simulink model "Copter"  (R2025a)
settings: Solver=ode1  StartTime=0.0  StopTime=inf  FixedStep=0.00125  RelTol=1e-3
libraries: aerolib6dof2 x4, AP_Conector_new x4
settings Model: PauseTimes=0:1  Creator=Peter  LastModifiedBy=danie
settings SolverCC: NumberNewtonIterations=2.0  AlgebraicLoopSolver=TrustRegion
settings DebuggingCC: UnconnectedInputMsg=warning  UnconnectedOutputMsg=warning  UnconnectedLineMsg=warning
settings ModelReferenceCC: EnableRefExpFcnMdlSchedulingChecks=on
settings RTWCC: GPUComputeCapability=3.5

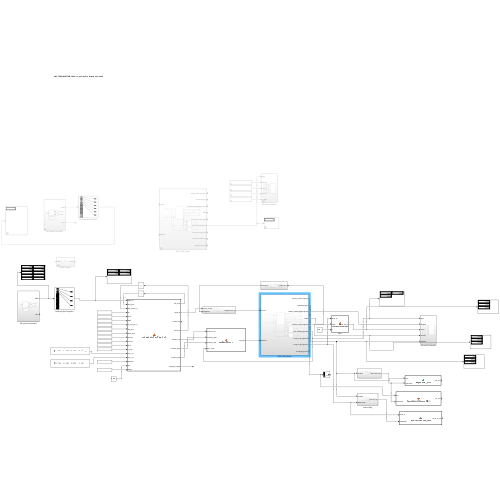
[thumbnail: Simulink's stored preview of the top-level diagram]
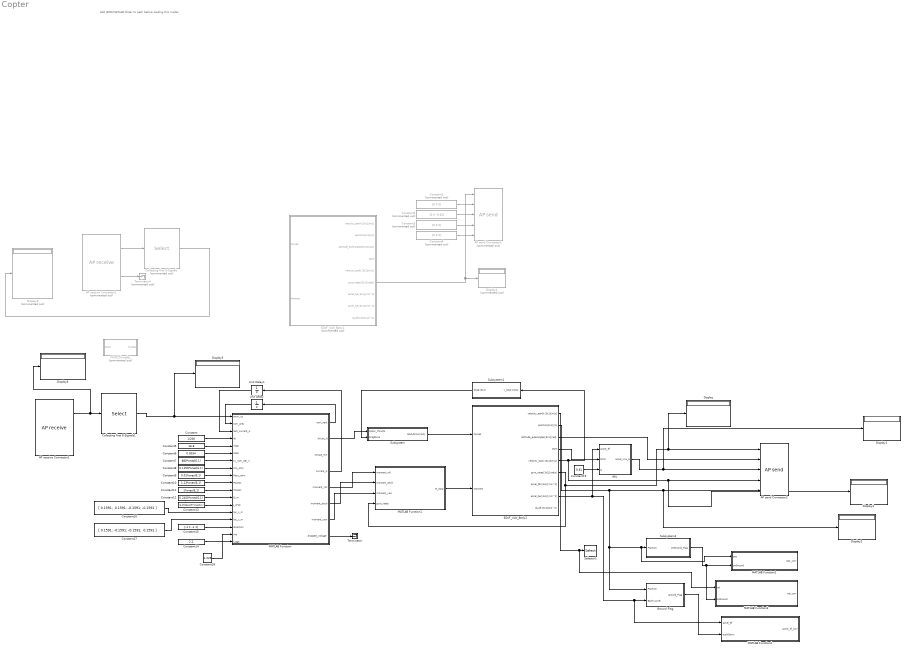
== system Copter ==
  note: Add JSON/MATLAB folder to path before loading this model
  6DoF_UAV_Body1 : Subsystem  Commented=on
  6DoF_UAV_Body2 : Subsystem
  AP receive Connector1 : AP_Conector_new/AP receive  Commented=on  SystemSampleTime=-1  VariantActivationTime=update diagram  EmptyChoice=off  PassThrough=off  PassThroughVariantControl=(default)  EmptyChoiceVariantControl=(default)  AllowFlexibleInterface=on  Latency=0  AutoFrameSizeCalculation=off
  AP receive Connector2 : AP_Conector_new/AP receive  SystemSampleTime=-1  VariantActivationTime=update diagram  EmptyChoice=off  PassThrough=off  PassThroughVariantControl=(default)  EmptyChoiceVariantControl=(default)  AllowFlexibleInterface=on  Latency=0  AutoFrameSizeCalculation=off
  AP send Connector1 : AP_Conector_new/AP send  Commented=on  SystemSampleTime=-1  VariantActivationTime=update diagram  EmptyChoice=off  PassThrough=off  PassThroughVariantControl=(default)  EmptyChoiceVariantControl=(default)  AllowFlexibleInterface=on  Latency=0  AutoFrameSizeCalculation=off
  AP send Connector2 : AP_Conector_new/AP send  SystemSampleTime=-1  VariantActivationTime=update diagram  EmptyChoice=off  PassThrough=off  PassThroughVariantControl=(default)  EmptyChoiceVariantControl=(default)  AllowFlexibleInterface=on  Latency=0  AutoFrameSizeCalculation=off
  Collecting first 6-Signals : Selector  Commented=on  InputPortWidth=16  IndexOptions=Index vector (dialog)  Indices=[1 2 3 4 5 6]  OutputSizes=1
  Collecting first 6-Signals1 : Selector  InputPortWidth=16  IndexOptions=Index vector (dialog)  Indices=[1 2 3 4]  OutputSizes=1
  Constant : Constant  Value=1/200
  Constant1 : Constant  Commented=on  Value=[0 0 0]
  Constant10 : Constant  Value=1.13*ones(6,1)
  Constant11 : Constant  Value=1*ones(6,1)
  Constant12 : Constant  Value=0.2450*ones(6,1)
  Constant13 : Constant  Value=(6.2526e-05)*ones(6,1)
  Constant14 : Constant  Value=2.2
  Constant15 : Constant  Value=[-1 1 -1 1]
  Constant16 : Constant  Value="[ 0.1591;  0.1591; -0.1591; -0.1591 ]"
  Constant17 : Constant  Value="[ 0.1591; -0.1591; -0.1591;  0.1591 ]"
  Constant18 : Constant  Value=1.225
  Constant19 : Constant  Value=9.81
  Constant2 : Constant  Commented=on  Value=[0 0 -9.81]
  Constant3 : Constant  Commented=on  Value=[0 0 0]
  Constant4 : Constant  Commented=on  Value=[0 0 0]
  Constant5 : Constant  Value=16.8
  Constant6 : Constant  Value=0.0034
  Constant7 : Constant  Value=880*ones(6,1)
  Constant8 : Constant  Value=0.1150*ones(6,1)
  Constant9 : Constant  Value=0.01*ones(6,1)
  Display{,1..3,5..6} (6 alike) : Display
  Display4 : Display  Commented=on
  Display9 : Display  Commented=on
  Ground Flag : Subsystem
  IMU : MATLAB Function  TreatAsAtomicUnit=on
  MATLAB Function : MATLAB Function  TreatAsAtomicUnit=on
  MATLAB Function1 : MATLAB Function  TreatAsAtomicUnit=on
  MATLAB Function2 : MATLAB Function  TreatAsAtomicUnit=on
  MATLAB Function3 : MATLAB Function  TreatAsAtomicUnit=on
  MATLAB Function4 : MATLAB Function  TreatAsAtomicUnit=on
  PWM2Throttle1 : Subsystem  Commented=on
  Selector1 : Selector  InputPortWidth=3  IndexOptions=Index vector (dialog)  Indices=[3]  OutputSizes=1
  Subsystem : Subsystem
  Subsystem1 : Subsystem
  Subsystem2 : Subsystem
  Terminator : Terminator
  Terminator4 : Terminator  Commented=on
  Unit Delay : UnitDelay  SampleTime=-1  HasFrameUpgradeWarning=on
  Unit Delay1 : UnitDelay  SampleTime=-1  HasFrameUpgradeWarning=on
  wires:
  Constant1/1 -> AP send Connector1/2
  Constant4/1 -> AP send Connector1/5
  Constant3/1 -> AP send Connector1/4
  Constant2/1 -> AP send Connector1/3
  AP receive Connector1/1 -> Collecting first 6-Signals/1
  AP receive Connector1/2 -> Terminator4/1
  Collecting first 6-Signals/1 -> Display9/1
  6DoF_UAV_Body1/6(gyro_rates[3x1][rad/s]) -> Display4/1, AP send Connector1/1
  MATLAB Function/1(rpm_next) -> Unit Delay/1
  Unit Delay/1 -> MATLAB Function/2(rpm_prev)
  AP receive Connector2/1 -> Display6/1, Collecting first 6-Signals1/1
  Constant/1 -> MATLAB Function/4(dt)
  Constant5/1 -> MATLAB Function/5(Vbat)
  Constant6/1 -> MATLAB Function/6(Rbat)
  Constant7/1 -> MATLAB Function/7(kv_rpm_per_V)
  Constant8/1 -> MATLAB Function/8(Rm_ohm)
  Constant9/1 -> MATLAB Function/9(Resc_ohm)
  Constant11/1 -> MATLAB Function/11(TConst)
  Constant10/1 -> MATLAB Function/10(PConst)
  Constant12/1 -> MATLAB Function/12(D_m)
  Constant13/1 -> MATLAB Function/13(J_prop)
  Constant14/1 -> MATLAB Function/18(fudge)
  MATLAB Function/4(current_A) -> Unit Delay1/1
  Unit Delay1/1 -> MATLAB Function/3(last_current_A)
  Constant15/1 -> MATLAB Function/16(direction)
  Constant16/1 -> MATLAB Function/14(loc_x_m)
  Constant17/1 -> MATLAB Function/15(loc_y_m)
  MATLAB Function/8(dropped_voltage) -> Terminator/1
  MATLAB Function/2(thrust_N) -> Subsystem/1(Motor_thrusts)
  Subsystem/1(Bodyforce [3x1]) -> 6DoF_UAV_Body2/1(Forces)
  6DoF_UAV_Body2/5(velocity_body [3x1][m/s]) -> Display3/1, AP send Connector2/4, Subsystem1/1(v_body [3x1])
  Subsystem1/1(Drag [3x1]) -> Subsystem/2(Dragforce)
  Constant18/1 -> MATLAB Function/17(rho)
  MATLAB Function1/1(M_body) -> 6DoF_UAV_Body2/2(Moment)
  MATLAB Function/5(moment_roll) -> MATLAB Function1/1(moment_roll)
  MATLAB Function/6(moment_pitch) -> MATLAB Function1/2(moment_pitch)
  MATLAB Function/7(moment_yaw) -> MATLAB Function1/3(moment_yaw)
  6DoF_UAV_Body2/6(gyro_rates[3x1][rad/s]) -> Display/1, AP send Connector2/1, MATLAB Function1/4(gyro_rates)
  6DoF_UAV_Body2/4(DCM) -> IMU/2(DCM)
  Constant19/1 -> IMU/3(g)
  6DoF_UAV_Body2/8(accel_be [3x1][m/s^2]) -> MATLAB Function4/1(accel_ef), Ground Flag/2(Earth Accel), IMU/1(accel_ef)
  IMU/1(accel_imu_b) -> Display1/1, AP send Connector2/3
  6DoF_UAV_Body2/3(attitude_eulerangles[3x1][rad]) -> AP send Connector2/2
  Collecting first 6-Signals1/1 -> Display5/1, MATLAB Function/1(pwm_us)
  6DoF_UAV_Body2/1(velocity_earth [3x1][m/s]) -> MATLAB Function3/1(vel), Selector1/1
  Ground Flag/1(ground_Flag) -> MATLAB Function4/2(pushDown)
  6DoF_UAV_Body2/2(position[3x1][m]) -> Ground Flag/1(Position), MATLAB Function2/1(pos), Subsystem2/1(Position), Display2/1, AP send Connector2/5
  Subsystem2/1(onGround_Flag) -> MATLAB Function3/2(onGround), MATLAB Function2/2(onGround)

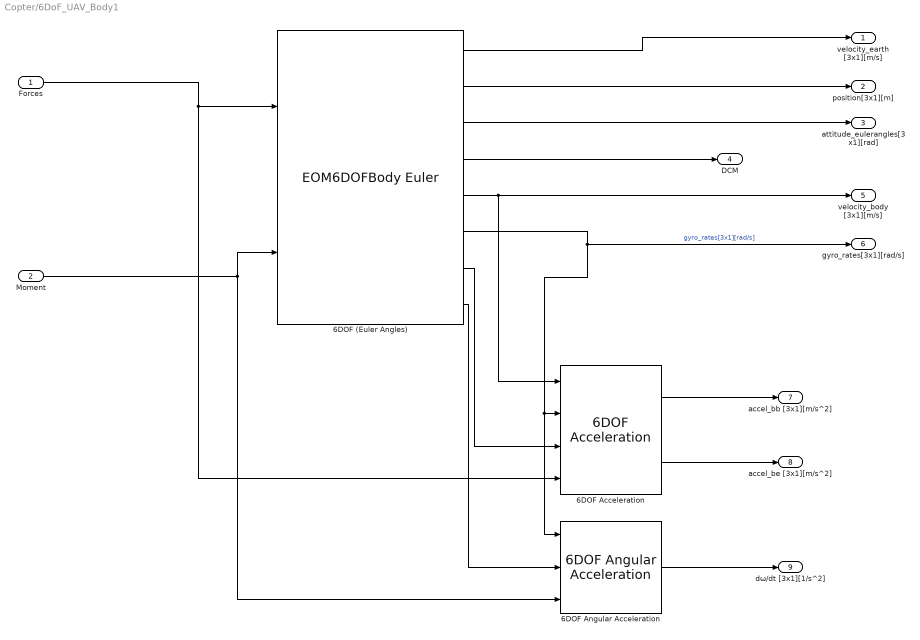
== system Copter/6DoF_UAV_Body1 ==
  Forces : Inport
  Moment : Inport  Port=2
  6DOF (Euler Angles) : EOM6DOFBodyEuler  mass_0=parameters.m  inertia=parameters.I  mass_flag=on
  6DOF Acceleration : aerolib6dof2/6DOF Acceleration  units=Metric (MKS)  mtype=Fixed  vre_flag=off
  6DOF Angular Acceleration : aerolib6dof2/6DOF Angular Acceleration  units=Metric (MKS)  mtype=Fixed
  velocity_earth [3x1][m/s] : Outport
  position[3x1][m] : Outport  Port=2
  attitude_eulerangles[3x1][rad] : Outport  Port=3
  DCM : Outport  Port=4
  velocity_body [3x1][m/s] : Outport  Port=5
  gyro_rates[3x1][rad/s] : Outport  Port=6
  accel_bb [3x1][m/s^2] : Outport  Port=7
  accel_be [3x1][m/s^2] : Outport  Port=8
  dω/dt [3x1][1/s^2] : Outport  Port=9
  wires:
  6DOF (Euler Angles)/3 -> attitude_eulerangles[3x1][rad]/1
  Moment/1 -> 6DOF (Euler Angles)/2, 6DOF Angular Acceleration/3
  6DOF Angular Acceleration/1 -> dω/dt [3x1][1/s^2]/1
  6DOF (Euler Angles)/6 -> gyro_rates[3x1][rad/s]/1, 6DOF Angular Acceleration/1, 6DOF Acceleration/2  "gyro_rates[3x1][rad/s]"
  6DOF Acceleration/2 -> accel_be [3x1][m/s^2]/1
  6DOF (Euler Angles)/5 -> velocity_body [3x1][m/s]/1, 6DOF Acceleration/1
  6DOF Acceleration/1 -> accel_bb [3x1][m/s^2]/1
  6DOF (Euler Angles)/8 -> 6DOF Angular Acceleration/2
  6DOF (Euler Angles)/7 -> 6DOF Acceleration/3
  6DOF (Euler Angles)/2 -> position[3x1][m]/1
  Forces/1 -> 6DOF Acceleration/4, 6DOF (Euler Angles)/1
  6DOF (Euler Angles)/1 -> velocity_earth [3x1][m/s]/1
  6DOF (Euler Angles)/4 -> DCM/1

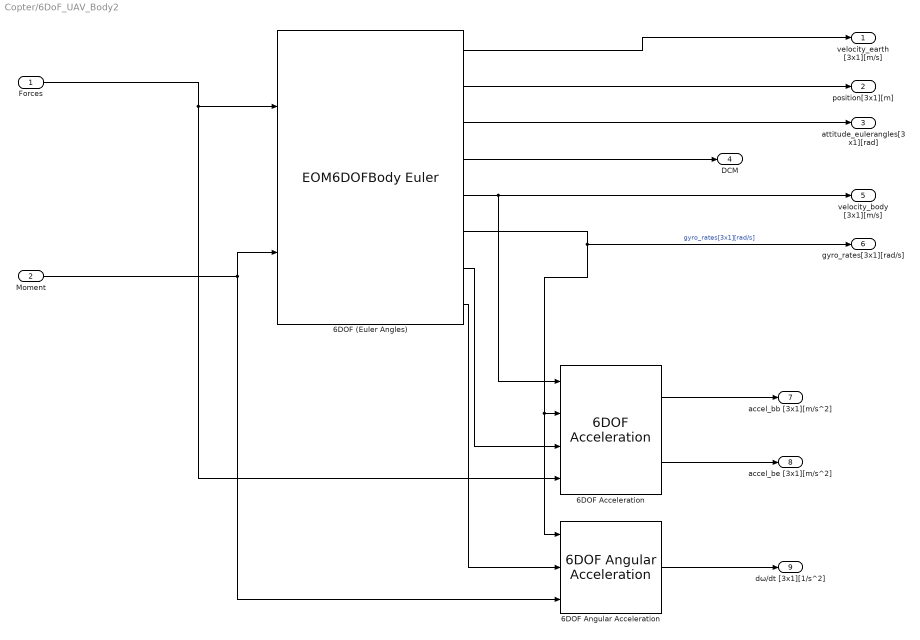
== system Copter/6DoF_UAV_Body2 ==
  Forces : Inport
  Moment : Inport  Port=2
  6DOF (Euler Angles) : EOM6DOFBodyEuler  mass_0=2  inertia=diag([0.0065 0.0065 0.0065])  mass_flag=on
  6DOF Acceleration : aerolib6dof2/6DOF Acceleration  units=Metric (MKS)  mtype=Fixed  vre_flag=off
  6DOF Angular Acceleration : aerolib6dof2/6DOF Angular Acceleration  units=Metric (MKS)  mtype=Fixed
  velocity_earth [3x1][m/s] : Outport
  position[3x1][m] : Outport  Port=2
  attitude_eulerangles[3x1][rad] : Outport  Port=3
  DCM : Outport  Port=4
  velocity_body [3x1][m/s] : Outport  Port=5
  gyro_rates[3x1][rad/s] : Outport  Port=6
  accel_bb [3x1][m/s^2] : Outport  Port=7
  accel_be [3x1][m/s^2] : Outport  Port=8
  dω/dt [3x1][1/s^2] : Outport  Port=9
  wires:
  6DOF (Euler Angles)/4 -> DCM/1
  6DOF (Euler Angles)/1 -> velocity_earth [3x1][m/s]/1
  Forces/1 -> 6DOF (Euler Angles)/1, 6DOF Acceleration/4
  6DOF (Euler Angles)/2 -> position[3x1][m]/1
  6DOF (Euler Angles)/7 -> 6DOF Acceleration/3
  6DOF (Euler Angles)/8 -> 6DOF Angular Acceleration/2
  6DOF Acceleration/1 -> accel_bb [3x1][m/s^2]/1
  6DOF (Euler Angles)/5 -> 6DOF Acceleration/1, velocity_body [3x1][m/s]/1
  6DOF Acceleration/2 -> accel_be [3x1][m/s^2]/1
  6DOF (Euler Angles)/6 -> 6DOF Acceleration/2, 6DOF Angular Acceleration/1, gyro_rates[3x1][rad/s]/1  "gyro_rates[3x1][rad/s]"
  6DOF Angular Acceleration/1 -> dω/dt [3x1][1/s^2]/1
  Moment/1 -> 6DOF Angular Acceleration/3, 6DOF (Euler Angles)/2
  6DOF (Euler Angles)/3 -> attitude_eulerangles[3x1][rad]/1

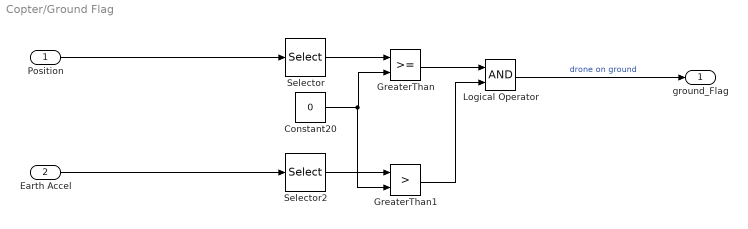
== system Copter/Ground Flag ==
  Position : Inport
  Earth Accel : Inport  Port=2
  Constant20 : Constant  Value=0
  GreaterThan : RelationalOperator  OutDataTypeStr=boolean  RndMeth=Simplest  InputSameDT=off
  GreaterThan1 : RelationalOperator  Operator=>  OutDataTypeStr=boolean  RndMeth=Simplest  InputSameDT=off
  Logical Operator : Logic  AllPortsSameDT=off  OutDataTypeStr=boolean
  Selector : Selector  InputPortWidth=3  IndexOptions=Index vector (dialog)  Indices=[3]  OutputSizes=1
  Selector2 : Selector  InputPortWidth=3  IndexOptions=Index vector (dialog)  Indices=[3]  OutputSizes=1
  ground_Flag : Outport
  wires:
  Selector2/1 -> GreaterThan1/1
  Selector/1 -> GreaterThan/1
  Constant20/1 -> GreaterThan1/2, GreaterThan/2
  Logical Operator/1 -> ground_Flag/1  "drone on ground"
  GreaterThan/1 -> Logical Operator/1
  GreaterThan1/1 -> Logical Operator/2
  Earth Accel/1 -> Selector2/1
  Position/1 -> Selector/1

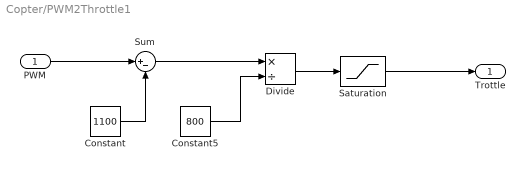
== system Copter/PWM2Throttle1 ==
  PWM : Inport
  Constant : Constant  Value=1100
  Constant5 : Constant  Value=800
  Divide : Product  Inputs=*/
  Saturation : Saturate  UpperLimit=1  LowerLimit=0
  Sum : Sum  Inputs=|+-
  Trottle : Outport
  wires:
  PWM/1 -> Sum/1
  Constant5/1 -> Divide/2
  Sum/1 -> Divide/1
  Divide/1 -> Saturation/1
  Constant/1 -> Sum/2
  Saturation/1 -> Trottle/1

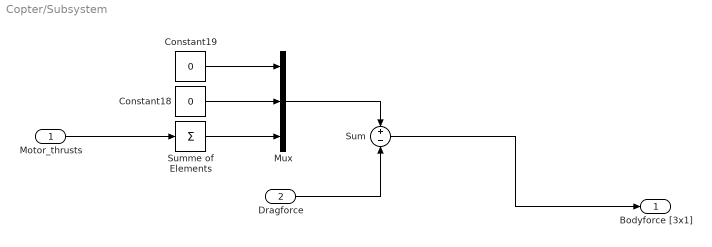
== system Copter/Subsystem ==
  Motor_thrusts : Inport
  Dragforce : Inport  Port=2
  Constant18 : Constant  Value=0
  Constant19 : Constant  Value=0
  Mux : Mux  Inputs=3
  Sum : Sum  Inputs=+-
  Summe of Elements : Sum  Inputs=+
  Bodyforce [3x1] : Outport
  wires:
  Constant19/1 -> Mux/1
  Sum/1 -> Bodyforce [3x1]/1
  Motor_thrusts/1 -> Summe of Elements/1
  Mux/1 -> Sum/1
  Dragforce/1 -> Sum/2
  Constant18/1 -> Mux/2
  Summe of Elements/1 -> Mux/3

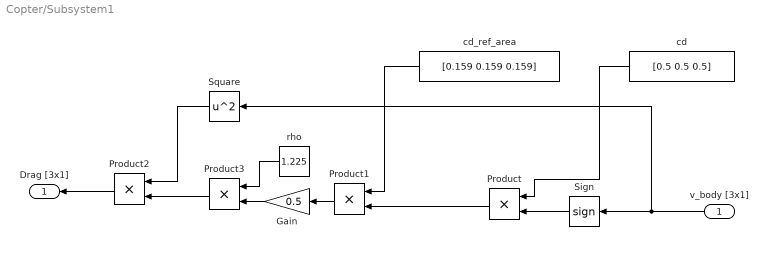
== system Copter/Subsystem1 ==
  v_body [3x1] : Inport
  Gain : Gain  Gain=0.5
  Product{,1..3} (4 alike) : Product
  Sign : Signum
  Square : Math  Operator=square
  cd : Constant  Value=[0.5 0.5 0.5]
  cd_ref_area : Constant  Value=[0.159 0.159 0.159]
  rho : Constant  Value=1.225
  Drag [3x1] : Outport
  wires:
  rho/1 -> Product3/1
  Gain/1 -> Product3/2
  Square/1 -> Product2/1
  cd/1 -> Product/1
  Product3/1 -> Product2/2
  v_body [3x1]/1 -> Square/1, Sign/1
  Sign/1 -> Product/2
  cd_ref_area/1 -> Product1/1
  Product/1 -> Product1/2
  Product1/1 -> Gain/1
  Product2/1 -> Drag [3x1]/1

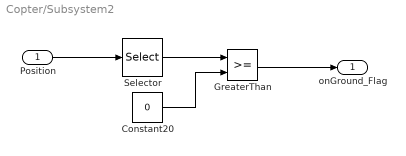
== system Copter/Subsystem2 ==
  Position : Inport
  Constant20 : Constant  Value=0
  GreaterThan : RelationalOperator  OutDataTypeStr=boolean  RndMeth=Simplest  InputSameDT=off
  Selector : Selector  InputPortWidth=3  IndexOptions=Index vector (dialog)  Indices=[3]  OutputSizes=1
  onGround_Flag : Outport
  wires:
  Constant20/1 -> GreaterThan/2
  GreaterThan/1 -> onGround_Flag/1
  Position/1 -> Selector/1
  Selector/1 -> GreaterThan/1

== matlab function Copter/MATLAB Function1 ==
  data: moment_roll input; M_body output; moment_pitch input; moment_yaw input; gyro_rates input
function M_body = buildBodyMoments(moment_roll, moment_pitch, moment_yaw, gyro_rates)
%#codegen
% moment_roll  [Mx1]  = T_i * x_i
% moment_pitch [Mx1]  = T_i * y_i
% moment_yaw   [Mx1]  = -Q_i * dir_i
% gyro_rates   [3x1]  = [p;q;r] rad/s (optional, for rotational drag)

% --- Sum motor contributions (SCRIPT-KONFORM)
Mx = -sum(moment_roll);
My =  sum(moment_pitch);
Mz =  sum(moment_yaw);

M_body = [Mx; My; Mz];

% --- Optional: rotational drag (wie im Script)
% rotational_drag = 0.2 * sign(gyro) .* gyro.^2;
if ~isempty(gyro_rates)
    rot_drag = 0.2 * sign(gyro_rates) .* (gyro_rates.^2);
    M_body = M_body - rot_drag;
end

end

== matlab function Copter/MATLAB Function ==
  data: pwm_us input; rpm_next output; rpm_prev input; last_current_A input; dt input; Vbat input; Rbat input; kv_rpm_per_V input; Rm_ohm input; Resc_ohm input; PConst input; TConst input; D_m input; J_prop input; loc_x_m input; loc_y_m input; direction input; rho input; fudge input; thrust_N output; torque_Nm output; current_A output; moment_roll output; moment_pitch output; moment_yaw output; dropped_voltage output
function [rpm_next, thrust_N, torque_Nm, current_A, ...
          moment_roll, moment_pitch, moment_yaw, dropped_voltage] = ...
    motorActuationFromPWM_1to1(pwm_us, rpm_prev, last_current_A, dt, ...
    Vbat, Rbat, ...
    kv_rpm_per_V, Rm_ohm, Resc_ohm, ...
    PConst, TConst, D_m, J_prop, ...
    loc_x_m, loc_y_m, direction, ...
    rho, fudge)
%#codegen
% 1:1 Logik wie im Jason/Hexsoon physics_step Motor-Loop

M = numel(pwm_us);

% Prealloc
rpm_next     = zeros(size(pwm_us));
thrust_N     = zeros(size(pwm_us));
torque_Nm    = zeros(size(pwm_us));
current_A    = zeros(size(pwm_us));
moment_roll  = zeros(size(pwm_us));
moment_pitch = zeros(size(pwm_us));
moment_yaw   = zeros(size(pwm_us));

% --- Battery sag (current draw from last step)
I_total = 0.0;
for i = 1:M
    I_total = I_total + last_current_A(i);
end
dropped_voltage = Vbat - Rbat * I_total;

% (Script macht keinen clamp; optional nur, wenn nötig)
% if dropped_voltage < 0, dropped_voltage = 0; end

two_pi = 2.0*pi;

for i = 1:M
    % --- throttle (0..1) from PWM
    throttle = (pwm_us(i) - 1100.0) / 800.0;
    if throttle < 0.0
        throttle = 0.0;
    elseif throttle > 1.0
        throttle = 1.0;
    end

    % effective voltage
    voltage = throttle * dropped_voltage;

    % Kt = 1 / (kv * (2*pi/60))
    kv = kv_rpm_per_V(i);
    if kv <= 1e-6
        kv = 1e-6;
    end
    Kt = 1.0 / (kv * (two_pi/60.0));

    % current = ((kv*voltage) - rpm) / ((Rtot)*kv)
    Rtot = Rm_ohm(i) + Resc_ohm(i);
    if Rtot <= 1e-6
        Rtot = 1e-6;
    end
    current = ((kv * voltage) - rpm_prev(i)) / (Rtot * kv);

    % torque = current * Kt
    torque = current * Kt;

    % prop_drag = PConst * rho * (rpm/60)^2 * D^5
    prop_drag = PConst(i) * rho * (rpm_prev(i)/60.0)^2 * (D_m(i)^5);

    % w = rpm*(2*pi/60)  [rad/s]
    w = rpm_prev(i) * (two_pi/60.0);

    % w1 = w + ((torque-prop_drag)/J) * dt
    J = J_prop(i);
    if J <= 1e-9
        J = 1e-9;
    end
    w1 = w + ((torque - prop_drag) / J) * dt;

    % rps = w1/(2*pi), clamp >=0
    rps = w1 * (1.0/two_pi);
    if rps < 0.0
        rps = 0.0;
    end

    % thrust = fudge * TConst * rho * rps^2 * D^4
    thrust = fudge * TConst(i) * rho * (rps*rps) * (D_m(i)^4);

    % moments
    m_roll  = thrust * loc_x_m(i);
    m_pitch = thrust * loc_y_m(i);
    m_yaw   = -torque * direction(i);

    % outputs
    current_A(i)    = current;
    torque_Nm(i)    = torque;
    rpm_next(i)     = rps * 60.0;
    thrust_N(i)     = thrust;
    moment_roll(i)  = m_roll;
    moment_pitch(i) = m_pitch;
    moment_yaw(i)   = m_yaw;
end
end

== matlab function Copter/IMU ==
  data: accel_ef input; accel_imu_b output; DCM input; g input
function accel_imu_b = kinematicToImuAccel(accel_ef, DCM, g)
%#codegen
% accel_ef: 3x1 kinematic accel in Earth frame (NED), without gravity
% DCM:      3x3 Body->Earth
% g:        scalar (m/s^2)

gvec_ef = [0; 0; -g];                 % NED: gravity is -g in Earth frame
accel_imu_b = DCM' * (accel_ef + gvec_ef);
end

== matlab function Copter/MATLAB Function2 ==
  data: pos input; pos_corr output; onGround input
function pos_corr = ClampPositionZ_NED(pos, onGround)
%#codegen
% Clamp Z-position (Down) to ground in NED coordinates

pos_corr = pos;

if onGround
    % NED: Down is positive, ground at z = 0
    pos_corr(3) = 0;
end

end

== matlab function Copter/MATLAB Function3 ==
  data: vel input; vel_corr output; onGround input
function vel_corr = ClampVelocityOnGround_NED(vel, onGround)
%#codegen
% Clamp velocity when drone is on ground (NED)

vel_corr = vel;

if onGround
    % MATLAB reference model: full velocity reset
    vel_corr(:) = 0;
end

end

== matlab function Copter/MATLAB Function4 ==
  data: accel_ef input; accel_ef_corr output; pushDown input
function accel_ef_corr = ClipAccelZPushDown_NED(accel_ef, pushDown)
%#codegen
% Clip downwards acceleration when pushing into the ground (NED)

accel_ef_corr = accel_ef;

if pushDown
    % NED: Down is positive
    accel_ef_corr(3) = 0;
end

end
